simulink model "Part5_"  (R2024a)
settings: Solver=VariableStepAuto  StartTime=0.0  StopTime=10.0  RelTol=1e-3
libraries: dspsrcs4 x1
settings Model: Creator=HP  LastModifiedBy=sujay

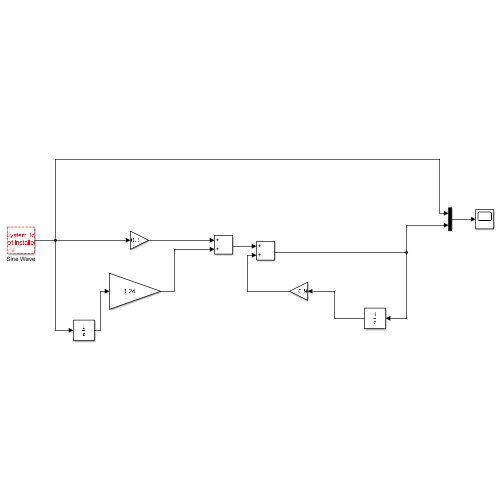
[thumbnail: Simulink's stored preview of the top-level diagram]
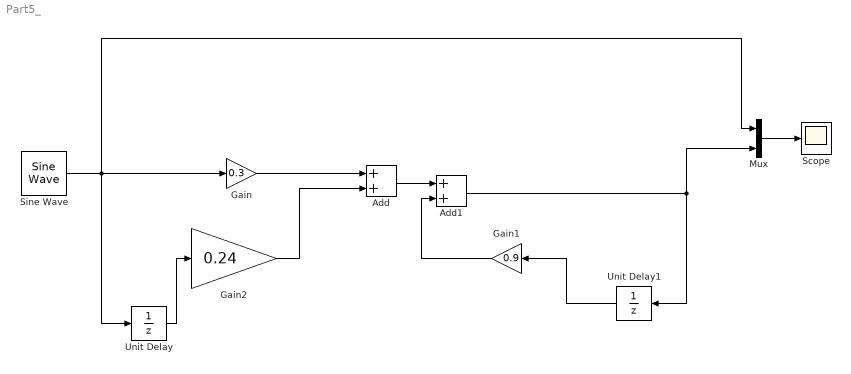
== system Part5_ ==
  Add : Sum
  Add1 : Sum
  Gain : Gain  Gain=0.3
  Gain1 : Gain  Gain=0.9
  Gain2 : Gain  Gain=0.24
  Mux : Mux  Inputs=2
  Scope : Scope
  Sine Wave : dspsrcs4/Sine Wave  Amplitude=1  Frequency=100  Phase=0  SampleMode=Discrete  OutComplex=Real  CompMethod=Trigonometric fcn  TableSize=Speed  SampleTime=1/1000  SamplesPerFrame=1  ResetState=Restart at time zero  OutputFrames=off  dataType=double  wordLen=16  udDataType=sfix(16)  fracBitsMode=Best precision  numFracBits=15  OutDataTypeStr=double  LastOutDataTypeStr=double
  Unit Delay : UnitDelay  SampleTime=-1  HasFrameUpgradeWarning=on
  Unit Delay1 : UnitDelay  SampleTime=-1  HasFrameUpgradeWarning=on
  wires:
  Sine Wave/1 -> Gain/1, Mux/1, Unit Delay/1
  Gain/1 -> Add/1
  Unit Delay/1 -> Gain2/1
  Gain2/1 -> Add/2
  Add/1 -> Add1/1
  Add1/1 -> Unit Delay1/1, Mux/2
  Unit Delay1/1 -> Gain1/1
  Gain1/1 -> Add1/2
  Mux/1 -> Scope/1
